simulink model "mass_spring_damper_sys"  (R2023a)
settings: Solver=VariableStepAuto  StartTime=0.0  StopTime=10.0  RelTol=1e-3
values from neighbouring files (symbols this model uses):
  b = 10    [model_script.m]
  k = 400    [model_script.m]
  m = massValue(i)    [model_script.m]
  x0 = 1    [model_script.m]
settings Model: Creator=EMRIX  LastModifiedBy=EMRIX

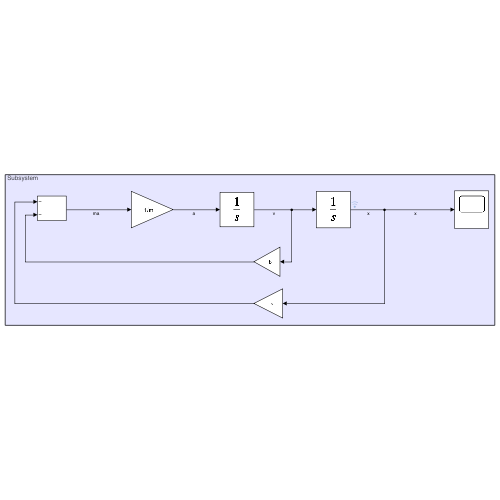
[thumbnail: Simulink's stored preview of the top-level diagram]
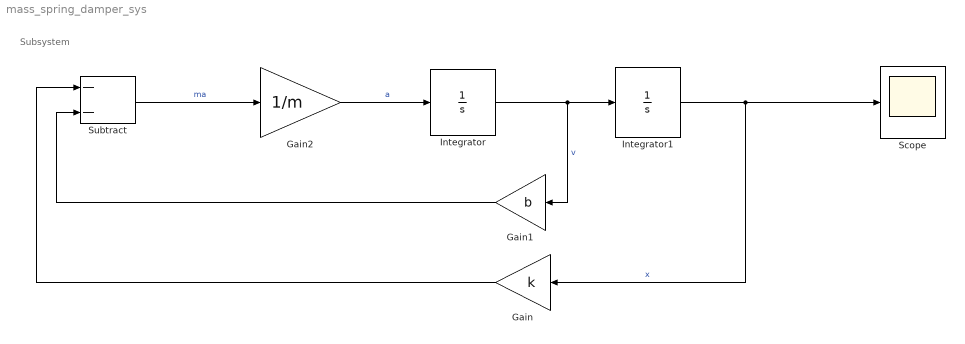
== system mass_spring_damper_sys ==
  note: Subsystem
  Gain : Gain  Gain=k
  Gain1 : Gain  Gain=b
  Gain2 : Gain  Gain=1/m
  Integrator : Integrator
  Integrator1 : Integrator  InitialCondition=x0
  Scope : Scope
  Subtract : Sum  Inputs=--
  wires:
  Gain2/1 -> Integrator/1  "a"
  Subtract/1 -> Gain2/1  "ma"
  Gain1/1 -> Subtract/2
  Gain/1 -> Subtract/1
  Integrator1/1 -> Gain/1, Scope/1  "x"
  Integrator/1 -> Integrator1/1, Gain1/1  "v"
